simulink model "revLimModel"  (R2017a)
settings: Solver=FixedStepDiscrete  StartTime=0.0  StopTime=3  FixedStep=0.001  RelTol=1e-3
undefined symbols (not defined in the file): GearRatios
libraries: simulink x8
settings Model: Creator=Johnny ZWall  LastModifiedBy=Johnny ZWall
settings DataIOCC: LimitDataPoints=on
settings OptimizationCC: DefaultParameterBehavior=Inlined  UseDivisionForNetSlopeComputation=on  UseFloatMulNetSlope=on  DefaultUnderspecifiedDataType=single  UseSpecifiedMinMax=on  InlineInvariantSignals=on  EnhancedBackFolding=on  CachingGlobalReferences=on  ZeroExternalMemoryAtStartup=off  ZeroInternalMemoryAtStartup=off  NoFixptDivByZeroProtection=on  EfficientFloat2IntCast=on  LifeSpan=inf  OptimizeBlockOrder=speed
settings DebuggingCC: ReadBeforeWriteMsg=EnableAllAsWarning  WriteAfterWriteMsg=EnableAllAsWarning  WriteAfterReadMsg=EnableAllAsWarning  IntegerOverflowMsg=error  UniqueDataStoreMsg=error  AllowSymbolicDim=off  NonBusSignalsTreatedAsBus=error  SFInvalidInputDataAccessInChartInitDiag=error  SFTransitionOutsideNaturalParentDiag=error  SFUnreachableExecutionPathDiag=error  SFUndirectedBroadcastEventsDiag=error  SFExecutionAtInitializationDiag=none  IntegerSaturationMsg=error
settings HardwareCC: ProdBitPerPointer=32  ProdBitPerSizeT=32  ProdBitPerPtrDiffT=32  ProdEndianess=BigEndian  ProdWordSize=32  ProdHWDeviceType=Renesas->SH-2/3/4
settings ModelReferenceCC: ModelReferenceNumInstancesAllowed=Single  PropagateSignalLabelsOutOfModel=off
settings SFSimCC: MATLABDynamicMemAlloc=off
settings RTWCC: SystemTargetFile=ert.tlc  GenCodeOnly=on  TemplateMakefile=ert_default_tmf  Description=Embedded Coder  BuildConfiguration=Faster Runs
settings RTWCC: CustomSourceCode=|
  | #include "EcuHacks.h"
  | 
  | D_Work rtDWork  __attribute__ ((section ("RamHole")));
settings CodeAppCC: GenerateComments=off  IgnoreCustomStorageClasses=off  CustomSymbolStrGlobalVar=rt$N$M  CustomSymbolStrType=$N$M  CustomSymbolStrFcn=$N$M$F  CustomSymbolStrMacro=$N$M  DefineNamingRule=LowerCase  ParamNamingRule=LowerCase  SignalNamingRule=LowerCase  SimulinkBlockComments=off  InternalIdentifier=Classic
settings ERTTargetCC: MultiwordLength=2048  IncludeMdlTerminateFcn=off  CombineSignalStateStructs=on  SuppressErrorStatus=on  SupportAbsoluteTime=off  SupportNonFinite=off  SupportComplex=off  CastingMode=Explicit  ExtModeTransport=2  ExtModeMexFile=sendToCommService  InlinedParameterPlacement=NonHierarchical  MultiInstanceErrorCode=None  RootIOFormat=Structure reference  ERTCustomFileTemplate=example_file_process.tlc  GlobalDataDefinition=InSourceFile  GlobalDataReference=InSourceFile  ERTFilePackagingFormat=Compact  PreserveExpressionOrder=on  PreserveIfCondition=on  IndentStyle=Allman
settings ConfigComp: CovMetricSettings=dw  CovHtmlReporting=on  CovSaveCumulativeToWorkspaceVar=on  CovSaveSingleToWorkspaceVar=on  CovExternalEMLEnable=off

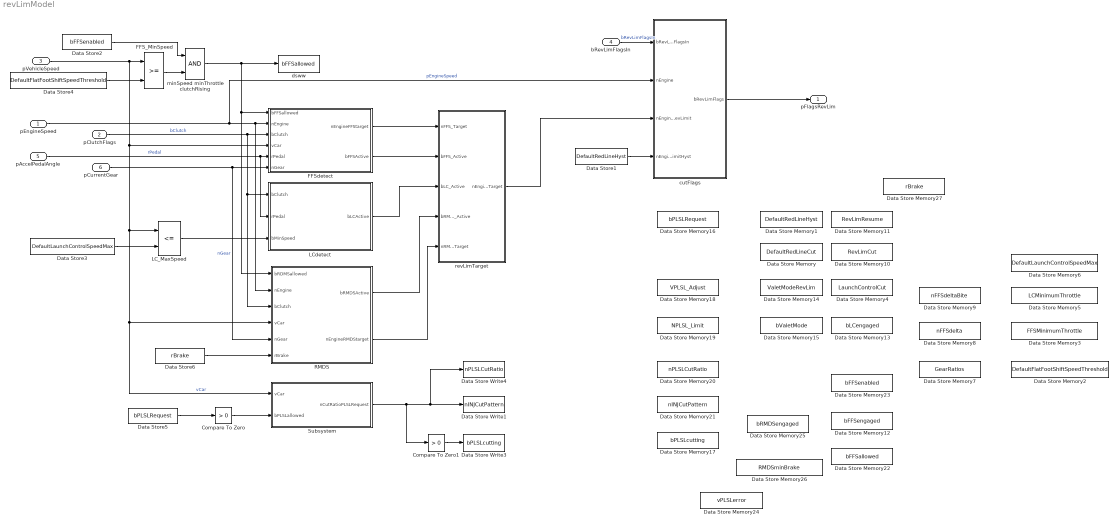
== system revLimModel ==
  pEngineSpeed : Inport  OutDataTypeStr=single  Interpolate=off
  pClutchFlags : Inport  Port=2  OutDataTypeStr=uint8
  pVehicleSpeed : Inport  Port=3  OutDataTypeStr=single
  bRevLimFlagsIn : Inport  Port=4  OutDataTypeStr=uint8
  pAccelPedalAngle : Inport  Port=5  OutDataTypeStr=single
  pCurrentGear : Inport  Port=6  OutDataTypeStr=uint8
  Compare To Zero : simulink/Logic and Bit Operations/Compare To Zero  relop=>  OutDataTypeStr=boolean
  Compare To Zero1 : simulink/Logic and Bit Operations/Compare To Zero  relop=>  OutDataTypeStr=boolean
  Data Store Memory : DataStoreMemory  DataStoreName=DefaultRedLineCut  InitialValue=6700  ShowAdditionalParam=off  OutDataTypeStr=single
  Data Store Memory1 : DataStoreMemory  DataStoreName=DefaultRedLineHyst  ReadBeforeWriteMsg=warning  WriteAfterWriteMsg=error  WriteAfterReadMsg=error  InitialValue=100  ShowAdditionalParam=off  OutDataTypeStr=single
  Data Store Memory10 : DataStoreMemory  DataStoreName=RevLimCut  ReadBeforeWriteMsg=warning  WriteAfterWriteMsg=warning  WriteAfterReadMsg=warning  InitialValue=2500  ShowAdditionalParam=off  OutDataTypeStr=single
  Data Store Memory11 : DataStoreMemory  DataStoreName=RevLimResume  ReadBeforeWriteMsg=warning  WriteAfterWriteMsg=warning  WriteAfterReadMsg=warning  InitialValue=2500  ShowAdditionalParam=off  OutDataTypeStr=single
  Data Store Memory12 : DataStoreMemory  DataStoreName=bFFSengaged  ReadBeforeWriteMsg=warning  WriteAfterWriteMsg=warning  WriteAfterReadMsg=warning  ShowAdditionalParam=off  OutDataTypeStr=boolean
  Data Store Memory13 : DataStoreMemory  DataStoreName=bLCengaged  ReadBeforeWriteMsg=warning  WriteAfterWriteMsg=warning  WriteAfterReadMsg=warning  ShowAdditionalParam=off  OutDataTypeStr=boolean
  Data Store Memory14 : DataStoreMemory  DataStoreName=ValetModeRevLim  InitialValue=4000  ShowAdditionalParam=off  OutDataTypeStr=single
  Data Store Memory15 : DataStoreMemory  DataStoreName=bValetMode  ReadBeforeWriteMsg=warning  WriteAfterWriteMsg=warning  WriteAfterReadMsg=warning  ShowAdditionalParam=off  OutDataTypeStr=uint8
  Data Store Memory16 : DataStoreMemory  DataStoreName=bPLSLRequest  ReadBeforeWriteMsg=warning  WriteAfterWriteMsg=warning  WriteAfterReadMsg=warning  ShowAdditionalParam=off  OutDataTypeStr=boolean
  Data Store Memory17 : DataStoreMemory  DataStoreName=bPLSLcutting  ReadBeforeWriteMsg=warning  WriteAfterWriteMsg=warning  WriteAfterReadMsg=warning  ShowAdditionalParam=off  OutDataTypeStr=boolean
  Data Store Memory18 : DataStoreMemory  DataStoreName=VPLSL_Adjust  ReadBeforeWriteMsg=warning  WriteAfterWriteMsg=warning  WriteAfterReadMsg=warning  ShowAdditionalParam=off  OutDataTypeStr=single
  Data Store Memory19 : DataStoreMemory  DataStoreName=NPLSL_Limit  ReadBeforeWriteMsg=warning  WriteAfterWriteMsg=warning  WriteAfterReadMsg=warning  InitialValue=25  ShowAdditionalParam=off  OutDataTypeStr=single
  Data Store Memory2 : DataStoreMemory  DataStoreName=DefaultFlatFootShiftSpeedThreshold  ReadBeforeWriteMsg=warning  WriteAfterWriteMsg=warning  WriteAfterReadMsg=warning  InitialValue=25  ShowAdditionalParam=off  OutDataTypeStr=single
  Data Store Memory20 : DataStoreMemory  DataStoreName=nPLSLCutRatio  ReadBeforeWriteMsg=warning  WriteAfterWriteMsg=warning  WriteAfterReadMsg=warning  ShowAdditionalParam=off  OutDataTypeStr=uint16
  Data Store Memory21 : DataStoreMemory  DataStoreName=nINJCutPattern  ReadBeforeWriteMsg=warning  WriteAfterWriteMsg=warning  WriteAfterReadMsg=warning  ShowAdditionalParam=off  OutDataTypeStr=uint16
  Data Store Memory22 : DataStoreMemory  DataStoreName=bFFSallowed  ReadBeforeWriteMsg=warning  WriteAfterWriteMsg=warning  WriteAfterReadMsg=warning  ShowAdditionalParam=off  OutDataTypeStr=boolean
  Data Store Memory23 : DataStoreMemory  DataStoreName=bFFSenabled  ReadBeforeWriteMsg=warning  WriteAfterWriteMsg=warning  WriteAfterReadMsg=warning  ShowAdditionalParam=off  OutDataTypeStr=boolean
  Data Store Memory24 : DataStoreMemory  DataStoreName=vPLSLerror  ReadBeforeWriteMsg=warning  WriteAfterWriteMsg=warning  WriteAfterReadMsg=warning  ShowAdditionalParam=off  OutDataTypeStr=single
  Data Store Memory25 : DataStoreMemory  DataStoreName=bRMDSengaged  ReadBeforeWriteMsg=warning  WriteAfterWriteMsg=warning  WriteAfterReadMsg=warning  ShowAdditionalParam=off  OutDataTypeStr=boolean
  Data Store Memory26 : DataStoreMemory  DataStoreName=RMDSminBrake  ReadBeforeWriteMsg=warning  WriteAfterWriteMsg=warning  WriteAfterReadMsg=warning  InitialValue=30  ShowAdditionalParam=off  OutDataTypeStr=single
  Data Store Memory27 : DataStoreMemory  DataStoreName=rBrake  ReadBeforeWriteMsg=warning  WriteAfterWriteMsg=warning  WriteAfterReadMsg=warning  InitialValue=23  ShowAdditionalParam=off  OutDataTypeStr=single
  Data Store Memory3 : DataStoreMemory  DataStoreName=FFSMinimumThrottle  ReadBeforeWriteMsg=warning  WriteAfterWriteMsg=warning  WriteAfterReadMsg=warning  InitialValue=85  ShowAdditionalParam=off  OutDataTypeStr=single
  Data Store Memory4 : DataStoreMemory  DataStoreName=LaunchControlCut  ReadBeforeWriteMsg=warning  WriteAfterWriteMsg=warning  WriteAfterReadMsg=warning  InitialValue=2500  ShowAdditionalParam=off  OutDataTypeStr=single
  Data Store Memory5 : DataStoreMemory  DataStoreName=LCMinimumThrottle  ReadBeforeWriteMsg=warning  WriteAfterWriteMsg=warning  WriteAfterReadMsg=warning  InitialValue=40  ShowAdditionalParam=off  OutDataTypeStr=single
  Data Store Memory6 : DataStoreMemory  DataStoreName=DefaultLaunchControlSpeedMax  ReadBeforeWriteMsg=warning  WriteAfterWriteMsg=warning  WriteAfterReadMsg=warning  InitialValue=3  ShowAdditionalParam=off  OutDataTypeStr=single
  Data Store Memory7 : DataStoreMemory  DataStoreName=GearRatios  ReadBeforeWriteMsg=warning  WriteAfterWriteMsg=warning  WriteAfterReadMsg=warning  InitialValue=[3.636,2.235,1.521,1.137,0.971,0.756]  ShowAdditionalParam=off  OutDataTypeStr=single  Dimensions=6
  Data Store Memory8 : DataStoreMemory  DataStoreName=nFFSdelta  ReadBeforeWriteMsg=warning  WriteAfterWriteMsg=warning  WriteAfterReadMsg=warning  InitialValue=300  ShowAdditionalParam=off  OutDataTypeStr=single
  Data Store Memory9 : DataStoreMemory  DataStoreName=nFFSdeltaBite  ReadBeforeWriteMsg=warning  WriteAfterWriteMsg=warning  WriteAfterReadMsg=warning  InitialValue=100  ShowAdditionalParam=off  OutDataTypeStr=single
  Data Store Write1 : DataStoreWrite  DataStoreName=nINJCutPattern
  Data Store Write3 : DataStoreWrite  DataStoreName=bPLSLcutting
  Data Store Write4 : DataStoreWrite  DataStoreName=nPLSLCutRatio
  Data Store1 : DataStoreRead  DataStoreName=DefaultRedLineHyst
  Data Store2 : DataStoreRead  DataStoreName=bFFSenabled  DataStoreElements=bFFSenabled
  Data Store3 : DataStoreRead  DataStoreName=DefaultLaunchControlSpeedMax
  Data Store4 : DataStoreRead  DataStoreName=DefaultFlatFootShiftSpeedThreshold
  Data Store5 : DataStoreRead  DataStoreName=bPLSLRequest  DataStoreElements=bPLSLRequest
  Data Store6 : DataStoreRead  DataStoreName=rBrake  DataStoreElements=rBrake
  FFS_MinSpeed : RelationalOperator  OutDataTypeStr=boolean  RndMeth=Nearest
  FFSdetect : Subsystem
  LC_MaxSpeed : RelationalOperator  Operator=<=  OutDataTypeStr=boolean  RndMeth=Nearest
  LCdetect : Subsystem
  RMDS : Subsystem
  Subsystem : Subsystem
  cutFlags : Subsystem
  dsww : DataStoreWrite  DataStoreName=bFFSallowed
  minSpeed minThrottle clutchRising : Logic  AllPortsSameDT=off  OutDataTypeStr=boolean
  revLimTarget : Subsystem
  pFlagsRevLim : Outport  SignalName=pFlagsRevLim  OutDataTypeStr=uint8
  wires:
  cutFlags/1(bRevLimFlags) -> pFlagsRevLim/1
  revLimTarget/1(nEngineTarget) -> cutFlags/3(nEngineRevLimit)
  pVehicleSpeed/1 -> FFSdetect/4(vCar), LC_MaxSpeed/1, RMDS/4(vCar), Subsystem/1(vCar), FFS_MinSpeed/1  "vCar"
  LC_MaxSpeed/1 -> LCdetect/3(bMinSpeed)
  minSpeed minThrottle clutchRising/1 -> dsww/1, FFSdetect/1(bFFSallowed), RMDS/1(bRDMSallowed)
  Data Store3/1 -> LC_MaxSpeed/2
  pCurrentGear/1 -> RMDS/5(nGear), FFSdetect/6(nGear)  "nGear"
  pAccelPedalAngle/1 -> LCdetect/2(rPedal), FFSdetect/5(rPedal)  "rPedal"
  Data Store4/1 -> FFS_MinSpeed/2
  Data Store1/1 -> cutFlags/4(nEngineCutLimitHyst)
  pClutchFlags/1 -> RMDS/3(bClutch), LCdetect/1(bClutch), FFSdetect/3(bClutch)  "bClutch"
  bRevLimFlagsIn/1 -> cutFlags/1(bRevLimFlagsIn)  "bRevLimFlagsIn"
  pEngineSpeed/1 -> cutFlags/2(nEngine), RMDS/2(nEngine), FFSdetect/2(nEngine)  "pEngineSpeed"
  FFSdetect/1(nEngineFFStarget) -> revLimTarget/1(nFFS_Target)
  FFSdetect/2(bFFSActive) -> revLimTarget/2(bFFS_Active)
  LCdetect/1(bLCActive) -> revLimTarget/3(bLC_Active)
  Data Store5/1 -> Compare To Zero/1
  Compare To Zero/1 -> Subsystem/2(bPLSLallowed)
  FFS_MinSpeed/1 -> minSpeed minThrottle clutchRising/2
  Data Store2/1 -> minSpeed minThrottle clutchRising/1
  Compare To Zero1/1 -> Data Store Write3/1
  Subsystem/1(nCutRatioPLSLRequest) -> Data Store Write4/1, Data Store Write1/1, Compare To Zero1/1
  Data Store6/1 -> RMDS/6(rBrake)
  RMDS/1(bRMDSActive) -> revLimTarget/4(bRMDS_Active)
  RMDS/2(nEngineRMDStarget) -> revLimTarget/5(nRMDS_Target)

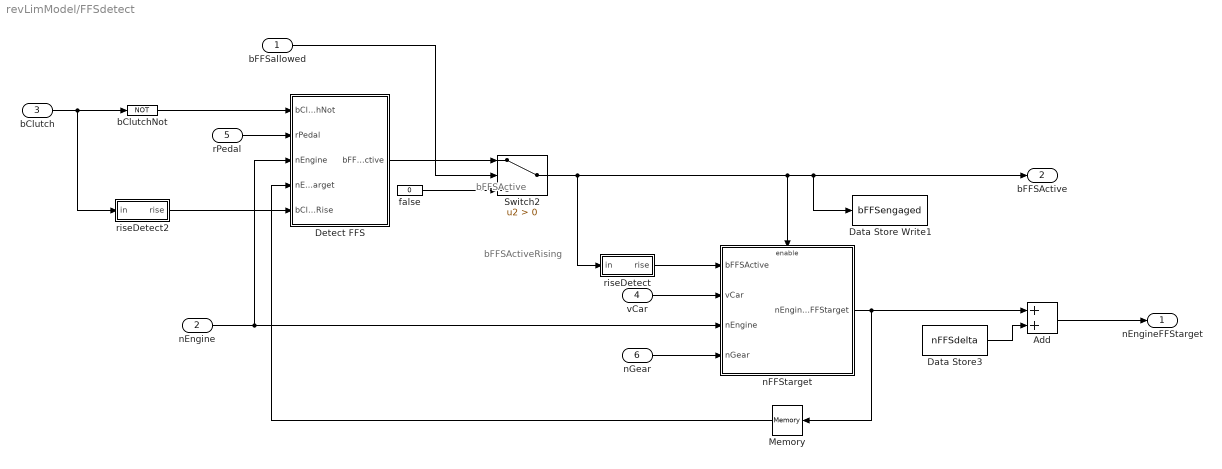
== system revLimModel/FFSdetect ==
  note: bFFSActiveRising
  note: bFFSActive
  bFFSallowed : Inport
  nEngine : Inport  Port=2
  bClutch : Inport  Port=3
  vCar : Inport  Port=4
  rPedal : Inport  Port=5
  nGear : Inport  Port=6
  Add : Sum
  Data Store Write1 : DataStoreWrite  DataStoreName=bFFSengaged
  Data Store3 : DataStoreRead  DataStoreName=nFFSdelta
  Detect FFS : Subsystem
  Memory : Memory
  Switch2 : Switch  Criteria=u2 > Threshold
  bClutchNot : Logic  Operator=NOT  AllPortsSameDT=off  OutDataTypeStr=boolean
  false : Constant  Value=0  OutDataTypeStr=boolean
  nFFStarget : Subsystem
      settings: RTWSystemCode=Inline
  riseDetect : Subsystem
  riseDetect2 : Subsystem
  nEngineFFStarget : Outport  InitialOutput=[0]
  bFFSActive : Outport  Port=2  OutputWhenDisabled=reset  InitialOutput=[0]
  wires:
  vCar/1 -> nFFStarget/2(vCar)
  nEngine/1 -> Detect FFS/3(nEngine), nFFStarget/3(nEngine)
  nGear/1 -> nFFStarget/4(nGear)
  nFFStarget/1(nEngineFFStarget) -> Memory/1, Add/1
  bClutch/1 -> bClutchNot/1, riseDetect2/1(in)
  rPedal/1 -> Detect FFS/2(rPedal)
  Switch2/1 -> riseDetect/1(in), Data Store Write1/1, bFFSActive/1, nFFStarget/Enable
  riseDetect/1(rise) -> nFFStarget/1(bFFSActive)
  Add/1 -> nEngineFFStarget/1
  Data Store3/1 -> Add/2
  Memory/1 -> Detect FFS/4(nEngineFFStarget)
  riseDetect2/1(rise) -> Detect FFS/5(bClutchRise)
  bClutchNot/1 -> Detect FFS/1(bClutchNot)
  Detect FFS/1(bFFSActive) -> Switch2/1
  bFFSallowed/1 -> Switch2/2
  false/1 -> Switch2/3

== system revLimModel/LCdetect ==
  bClutch : Inport
  rPedal : Inport  Port=2
  bMinSpeed : Inport  Port=3
  Data Store3 : DataStoreRead  DataStoreName=LCMinimumThrottle
  LC_MinPedal : RelationalOperator  OutDataTypeStr=boolean  RndMeth=Nearest
  maxSpeed minThrottle clutchRising : Logic  Inputs=3  AllPortsSameDT=off  OutDataTypeStr=boolean
  bLCActive : Outport  OutputWhenDisabled=reset  InitialOutput=[0]
  wires:
  Data Store3/1 -> LC_MinPedal/2
  rPedal/1 -> LC_MinPedal/1
  maxSpeed minThrottle clutchRising/1 -> bLCActive/1  "bLCstateSet"
  LC_MinPedal/1 -> maxSpeed minThrottle clutchRising/3  "bLCrPedakOK"
  bClutch/1 -> maxSpeed minThrottle clutchRising/2  "bClutchFalling"
  bMinSpeed/1 -> maxSpeed minThrottle clutchRising/1

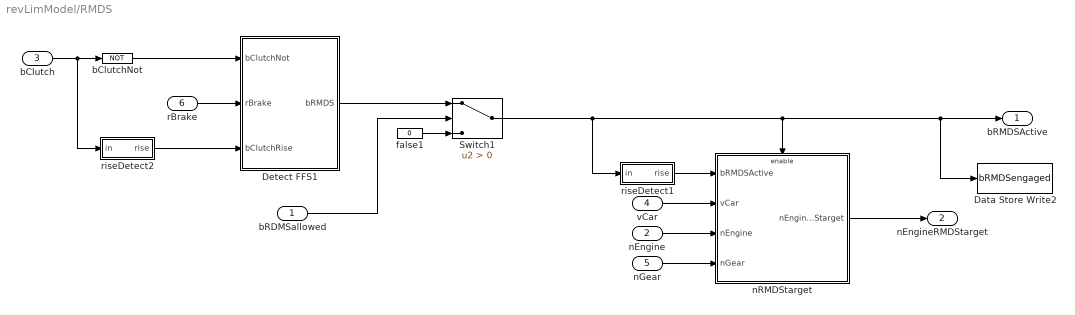
== system revLimModel/RMDS ==
  bRDMSallowed : Inport
  nEngine : Inport  Port=2
  bClutch : Inport  Port=3
  vCar : Inport  Port=4
  nGear : Inport  Port=5
  rBrake : Inport  Port=6
  Data Store Write2 : DataStoreWrite  DataStoreName=bRMDSengaged
  Detect FFS1 : Subsystem
  Switch1 : Switch  Criteria=u2 > Threshold
  bClutchNot : Logic  Operator=NOT  AllPortsSameDT=off  OutDataTypeStr=boolean
  false1 : Constant  Value=0  OutDataTypeStr=boolean
  nRMDStarget : Subsystem
      settings: RTWSystemCode=Inline
  riseDetect1 : Subsystem
  riseDetect2 : Subsystem
  bRMDSActive : Outport  OutputWhenDisabled=reset  InitialOutput=[0]
  nEngineRMDStarget : Outport  Port=2  InitialOutput=[0]
  wires:
  vCar/1 -> nRMDStarget/2(vCar)
  nEngine/1 -> nRMDStarget/3(nEngine)
  nGear/1 -> nRMDStarget/4(nGear)
  bClutch/1 -> bClutchNot/1, riseDetect2/1(in)
  rBrake/1 -> Detect FFS1/2(rBrake)
  Switch1/1 -> Data Store Write2/1, bRMDSActive/1, nRMDStarget/Enable, riseDetect1/1(in)
  nRMDStarget/1(nEngineRMDStarget) -> nEngineRMDStarget/1
  riseDetect1/1(rise) -> nRMDStarget/1(bRMDSActive)
  riseDetect2/1(rise) -> Detect FFS1/3(bClutchRise)
  bClutchNot/1 -> Detect FFS1/1(bClutchNot)
  Detect FFS1/1(bRMDS) -> Switch1/1
  bRDMSallowed/1 -> Switch1/2
  false1/1 -> Switch1/3

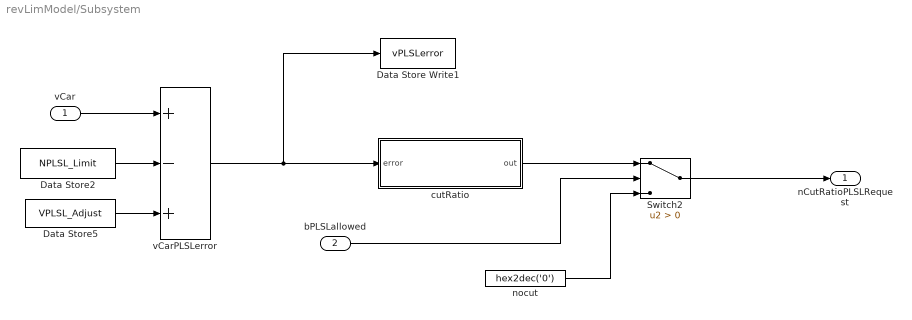
== system revLimModel/Subsystem ==
  vCar : Inport
  bPLSLallowed : Inport  Port=2
  Data Store Write1 : DataStoreWrite  DataStoreName=vPLSLerror  DataStoreElements=vPLSLerror
  Data Store2 : DataStoreRead  DataStoreName=NPLSL_Limit
  Data Store5 : DataStoreRead  DataStoreName=VPLSL_Adjust  DataStoreElements=VPLSL_Adjust
  Switch2 : Switch  Criteria=u2 > Threshold
  cutRatio : Subsystem
  nocut : Constant  Value=hex2dec('0')  OutDataTypeStr=uint16
  vCarPLSLerror : Sum  Inputs=+-+
  nCutRatioPLSLRequest : Outport  OutDataTypeStr=uint16  OutputWhenDisabled=reset  InitialOutput=[0]
  wires:
  Data Store2/1 -> vCarPLSLerror/2
  vCar/1 -> vCarPLSLerror/1
  Data Store5/1 -> vCarPLSLerror/3
  vCarPLSLerror/1 -> Data Store Write1/1, cutRatio/1(error)
  cutRatio/1(out) -> Switch2/1
  Switch2/1 -> nCutRatioPLSLRequest/1
  bPLSLallowed/1 -> Switch2/2
  nocut/1 -> Switch2/3

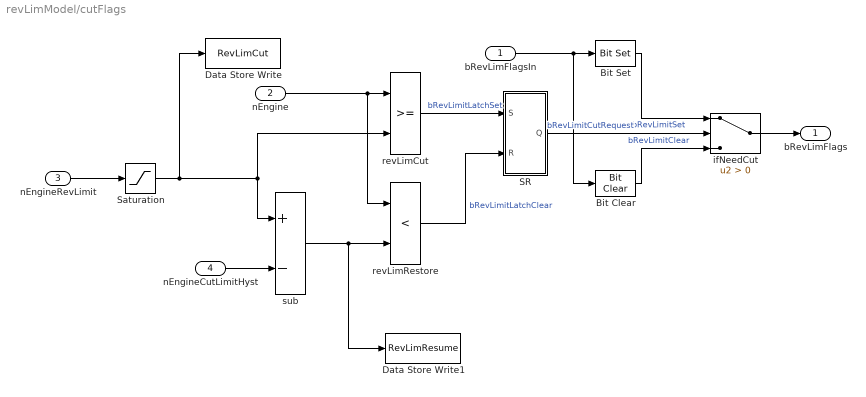
== system revLimModel/cutFlags ==
  bRevLimFlagsIn : Inport  OutDataTypeStr=uint8
  nEngine : Inport  Port=2
  nEngineRevLimit : Inport  Port=3
  nEngineCutLimitHyst : Inport  Port=4
  Bit Clear : simulink/Logic and Bit Operations/Bit Clear  iBit=0
      settings: SourceProductName=Simulink  SourceProductBaseCode=SL
  Bit Set : simulink/Logic and Bit Operations/Bit Set  iBit=0
      settings: SourceProductName=Simulink  SourceProductBaseCode=SL
  Data Store Write : DataStoreWrite  DataStoreName=RevLimCut
  Data Store Write1 : DataStoreWrite  DataStoreName=RevLimResume
  SR : Subsystem
  Saturation : Saturate  UpperLimit=6800  LowerLimit=2100
  ifNeedCut : Switch  Criteria=u2 > Threshold
  revLimCut : RelationalOperator  OutDataTypeStr=boolean  RndMeth=Nearest
  revLimRestore : RelationalOperator  Operator=<  OutDataTypeStr=boolean  RndMeth=Nearest
  sub : Sum  Inputs=+-
  bRevLimFlags : Outport
  wires:
  Bit Clear/1 -> ifNeedCut/3  "bRevLimitClear"
  nEngineCutLimitHyst/1 -> sub/2
  nEngine/1 -> revLimRestore/1, revLimCut/1
  sub/1 -> Data Store Write1/1, revLimRestore/2
  ifNeedCut/1 -> bRevLimFlags/1
  revLimCut/1 -> SR/1(S)  "bRevLimitLatchSet"
  bRevLimFlagsIn/1 -> Bit Clear/1, Bit Set/1
  revLimRestore/1 -> SR/2(R)  "bRevLimitLatchClear"
  Bit Set/1 -> ifNeedCut/1  "bRevLimitSet"
  SR/1(Q) -> ifNeedCut/2  "bRevLimitCutRequest"
  Saturation/1 -> Data Store Write/1, sub/1, revLimCut/2
  nEngineRevLimit/1 -> Saturation/1

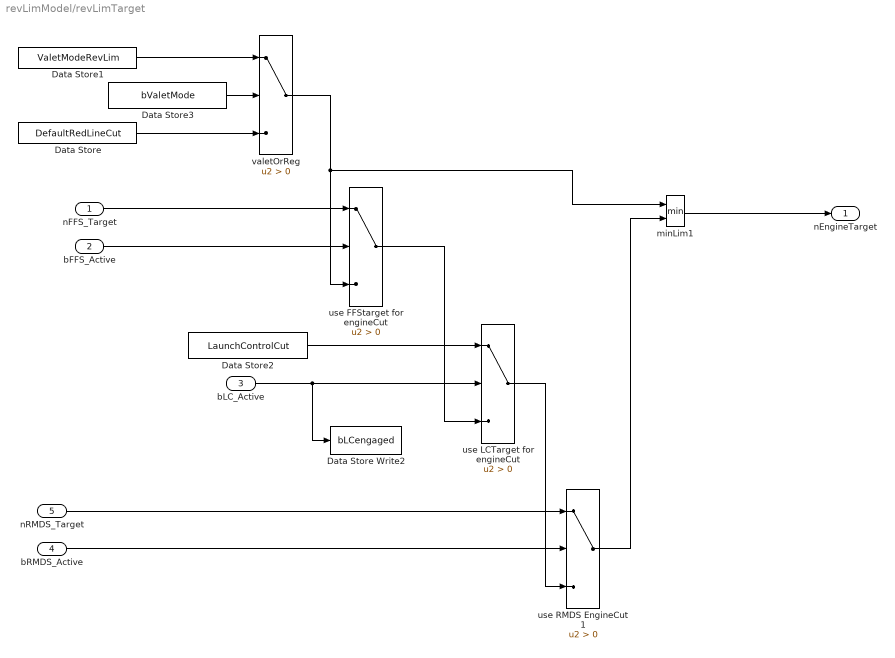
== system revLimModel/revLimTarget ==
  nFFS_Target : Inport
  bFFS_Active : Inport  Port=2
  bLC_Active : Inport  Port=3
  bRMDS_Active : Inport  Port=4
  nRMDS_Target : Inport  Port=5
  Data Store : DataStoreRead  DataStoreName=DefaultRedLineCut
  Data Store Write2 : DataStoreWrite  DataStoreName=bLCengaged
  Data Store1 : DataStoreRead  DataStoreName=ValetModeRevLim
  Data Store2 : DataStoreRead  DataStoreName=LaunchControlCut  DataStoreElements=LaunchControlCut
  Data Store3 : DataStoreRead  DataStoreName=bValetMode  DataStoreElements=bValetMode
  minLim1 : MinMax  Inputs=2  OutDataTypeStr=single
  use FFStarget for engineCut : Switch  Criteria=u2 > Threshold  OutDataTypeStr=single
  use LCTarget for engineCut : Switch  Criteria=u2 > Threshold  OutDataTypeStr=single
  use RMDS EngineCut1 : Switch  Criteria=u2 > Threshold  OutDataTypeStr=single
  valetOrReg : Switch  Criteria=u2 > Threshold  OutDataTypeStr=single
  nEngineTarget : Outport
  wires:
  bLC_Active/1 -> Data Store Write2/1, use LCTarget for engineCut/2
  use RMDS EngineCut1/1 -> minLim1/2
  bFFS_Active/1 -> use FFStarget for engineCut/2
  valetOrReg/1 -> minLim1/1, use FFStarget for engineCut/3
  use FFStarget for engineCut/1 -> use LCTarget for engineCut/3
  Data Store2/1 -> use LCTarget for engineCut/1
  nFFS_Target/1 -> use FFStarget for engineCut/1
  minLim1/1 -> nEngineTarget/1
  Data Store/1 -> valetOrReg/3
  Data Store1/1 -> valetOrReg/1
  Data Store3/1 -> valetOrReg/2
  nRMDS_Target/1 -> use RMDS EngineCut1/1
  bRMDS_Active/1 -> use RMDS EngineCut1/2
  use LCTarget for engineCut/1 -> use RMDS EngineCut1/3

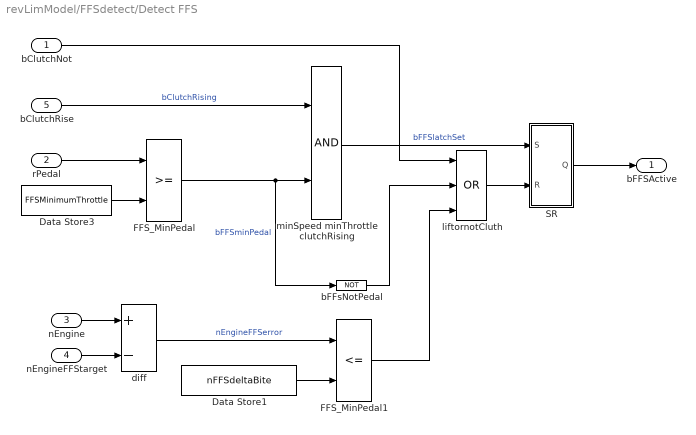
== system revLimModel/FFSdetect/Detect FFS ==
  bClutchNot : Inport
  rPedal : Inport  Port=2
  nEngine : Inport  Port=3
  nEngineFFStarget : Inport  Port=4
  bClutchRise : Inport  Port=5
  Data Store1 : DataStoreRead  DataStoreName=nFFSdeltaBite
  Data Store3 : DataStoreRead  DataStoreName=FFSMinimumThrottle
  FFS_MinPedal : RelationalOperator  OutDataTypeStr=boolean  RndMeth=Nearest
  FFS_MinPedal1 : RelationalOperator  Operator=<=  OutDataTypeStr=boolean  RndMeth=Nearest
  SR : Subsystem
  bFFsNotPedal : Logic  Operator=NOT  AllPortsSameDT=off  OutDataTypeStr=boolean
  diff : Sum  Inputs=+-
  "liftornotCluth " : Logic  Operator=OR  Inputs=3  AllPortsSameDT=off  OutDataTypeStr=boolean
  minSpeed minThrottle clutchRising : Logic  AllPortsSameDT=off  OutDataTypeStr=boolean
  bFFSActive : Outport
  wires:
  Data Store3/1 -> FFS_MinPedal/2
  rPedal/1 -> FFS_MinPedal/1
  bClutchRise/1 -> minSpeed minThrottle clutchRising/1  "bClutchRising"
  SR/1(Q) -> bFFSActive/1
  minSpeed minThrottle clutchRising/1 -> SR/1(S)  "bFFSlatchSet"
  FFS_MinPedal/1 -> bFFsNotPedal/1, minSpeed minThrottle clutchRising/2  "bFFSminPedal"
  bClutchNot/1 -> "liftornotCluth "/1
  "liftornotCluth "/1 -> SR/2(R)
  bFFsNotPedal/1 -> "liftornotCluth "/2
  nEngine/1 -> diff/1
  nEngineFFStarget/1 -> diff/2
  diff/1 -> FFS_MinPedal1/1  "nEngineFFSerror"
  Data Store1/1 -> FFS_MinPedal1/2
  FFS_MinPedal1/1 -> "liftornotCluth "/3

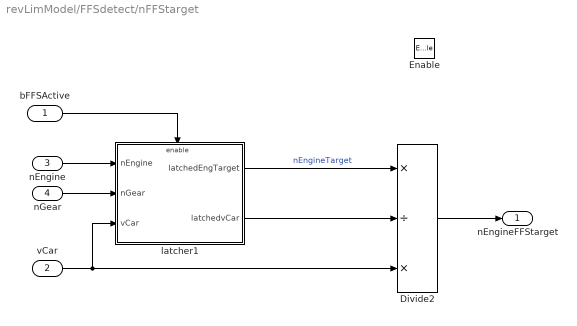
== system revLimModel/FFSdetect/nFFStarget ==
  bFFSActive : Inport
  vCar : Inport  Port=2
  nEngine : Inport  Port=3
  nGear : Inport  Port=4
  Enable : EnablePort
  Divide2 : Product  Inputs=*/*
  latcher1 : Subsystem
  nEngineFFStarget : Outport
  wires:
  Divide2/1 -> nEngineFFStarget/1
  vCar/1 -> Divide2/3, latcher1/3(vCar)
  latcher1/1(latchedEngTarget) -> Divide2/1  "nEngineTarget"
  bFFSActive/1 -> latcher1/Enable
  nGear/1 -> latcher1/2(nGear)
  latcher1/2(latchedvCar) -> Divide2/2
  nEngine/1 -> latcher1/1(nEngine)

== system revLimModel/FFSdetect/riseDetect ==
  in : Inport
  Memory : Memory
  rising : RelationalOperator  Operator=>  OutDataTypeStr=boolean  RndMeth=Simplest
  rise : Outport
  wires:
  Memory/1 -> rising/2
  in/1 -> rising/1, Memory/1
  rising/1 -> rise/1

== system revLimModel/FFSdetect/riseDetect2 ==
  in : Inport
  Memory : Memory
  rising : RelationalOperator  Operator=>  OutDataTypeStr=boolean  RndMeth=Simplest
  rise : Outport
  wires:
  Memory/1 -> rising/2
  in/1 -> rising/1, Memory/1
  rising/1 -> rise/1

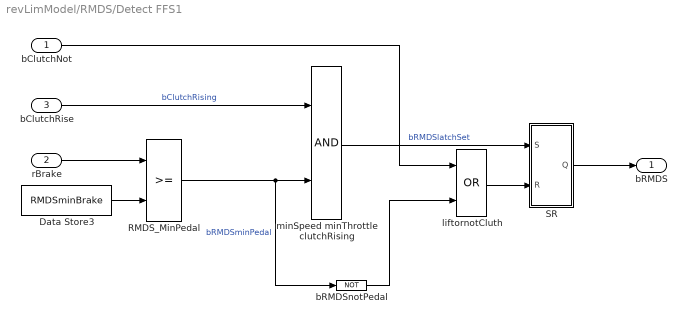
== system revLimModel/RMDS/Detect FFS1 ==
  bClutchNot : Inport
  rBrake : Inport  Port=2
  bClutchRise : Inport  Port=3
  Data Store3 : DataStoreRead  DataStoreName=RMDSminBrake
  RMDS_MinPedal : RelationalOperator  OutDataTypeStr=boolean  RndMeth=Nearest
  SR : Subsystem
  bRMDSnotPedal : Logic  Operator=NOT  AllPortsSameDT=off  OutDataTypeStr=boolean
  "liftornotCluth " : Logic  Operator=OR  AllPortsSameDT=off  OutDataTypeStr=boolean
  minSpeed minThrottle clutchRising : Logic  AllPortsSameDT=off  OutDataTypeStr=boolean
  bRMDS : Outport
  wires:
  Data Store3/1 -> RMDS_MinPedal/2
  rBrake/1 -> RMDS_MinPedal/1
  bClutchRise/1 -> minSpeed minThrottle clutchRising/1  "bClutchRising"
  SR/1(Q) -> bRMDS/1
  minSpeed minThrottle clutchRising/1 -> SR/1(S)  "bRMDSlatchSet"
  RMDS_MinPedal/1 -> bRMDSnotPedal/1, minSpeed minThrottle clutchRising/2  "bRMDSminPedal"
  bClutchNot/1 -> "liftornotCluth "/1
  "liftornotCluth "/1 -> SR/2(R)
  bRMDSnotPedal/1 -> "liftornotCluth "/2

== system revLimModel/RMDS/nRMDStarget ==
  bRMDSActive : Inport
  vCar : Inport  Port=2
  nEngine : Inport  Port=3
  nGear : Inport  Port=4
  Enable : EnablePort
  Divide2 : Product  Inputs=*/*
  latcher1 : Subsystem
  nEngineRMDStarget : Outport
  wires:
  Divide2/1 -> nEngineRMDStarget/1
  vCar/1 -> Divide2/3, latcher1/3(vCar)
  latcher1/1(latchedEngTarget) -> Divide2/1  "nEngineTarget"
  bRMDSActive/1 -> latcher1/Enable
  nGear/1 -> latcher1/2(nGear)
  latcher1/2(latchedvCar) -> Divide2/2
  nEngine/1 -> latcher1/1(nEngine)

== system revLimModel/RMDS/riseDetect1 ==
  in : Inport
  Memory : Memory
  rising : RelationalOperator  Operator=>  OutDataTypeStr=boolean  RndMeth=Simplest
  rise : Outport
  wires:
  Memory/1 -> rising/2
  in/1 -> rising/1, Memory/1
  rising/1 -> rise/1

== system revLimModel/RMDS/riseDetect2 ==
  in : Inport
  Memory : Memory
  rising : RelationalOperator  Operator=>  OutDataTypeStr=boolean  RndMeth=Simplest
  rise : Outport
  wires:
  Memory/1 -> rising/2
  in/1 -> rising/1, Memory/1
  rising/1 -> rise/1

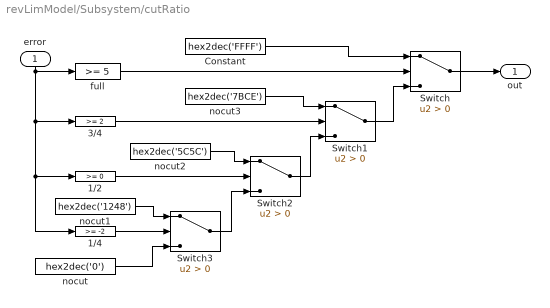
== system revLimModel/Subsystem/cutRatio ==
  error : Inport
  1/2 : simulink/Logic and Bit Operations/Compare To Constant  relop=>=  const=0  OutDataTypeStr=boolean
  1/4 : simulink/Logic and Bit Operations/Compare To Constant  relop=>=  const=-2  OutDataTypeStr=boolean
  3/4 : simulink/Logic and Bit Operations/Compare To Constant  relop=>=  const=2  OutDataTypeStr=boolean
  Constant : Constant  Value=hex2dec('FFFF')  OutDataTypeStr=uint16
  Switch{,1..3} (4 alike) : Switch  Criteria=u2 > Threshold
  full : simulink/Logic and Bit Operations/Compare To Constant  relop=>=  const=5  OutDataTypeStr=boolean
  nocut : Constant  Value=hex2dec('0')  OutDataTypeStr=uint16
  nocut1 : Constant  Value=hex2dec('1248')  OutDataTypeStr=uint16
  nocut2 : Constant  Value=hex2dec('5C5C')  OutDataTypeStr=uint16
  nocut3 : Constant  Value=hex2dec('7BCE')  OutDataTypeStr=uint16
  out : Outport
  wires:
  nocut1/1 -> Switch3/1
  1/2/1 -> Switch2/2
  Switch2/1 -> Switch1/3
  1/4/1 -> Switch3/2
  3/4/1 -> Switch1/2
  Switch/1 -> out/1
  full/1 -> Switch/2
  Switch3/1 -> Switch2/3
  error/1 -> full/1, 3/4/1, 1/2/1, 1/4/1
  nocut/1 -> Switch3/3
  nocut3/1 -> Switch1/1
  Switch1/1 -> Switch/3
  Constant/1 -> Switch/1
  nocut2/1 -> Switch2/1

== system revLimModel/cutFlags/SR ==
  S : Inport
  R : Inport  Port=2
  mem : Memory
  notMem : Logic  Operator=NOT  AllPortsSameDT=off  OutDataTypeStr=boolean
  reset : Logic  Operator=NOR  AllPortsSameDT=off  OutDataTypeStr=boolean
  set : Logic  Operator=OR  AllPortsSameDT=off  OutDataTypeStr=boolean
  Q : Outport
  wires:
  S/1 -> set/1
  set/1 -> mem/1, Q/1
  reset/1 -> set/2
  mem/1 -> notMem/1
  notMem/1 -> reset/1
  R/1 -> reset/2

== system revLimModel/FFSdetect/Detect FFS/SR ==
  S : Inport
  R : Inport  Port=2
  mem : Memory
  notMem : Logic  Operator=NOT  AllPortsSameDT=off  OutDataTypeStr=boolean
  reset : Logic  Operator=NOR  AllPortsSameDT=off  OutDataTypeStr=boolean
  set : Logic  Operator=OR  AllPortsSameDT=off  OutDataTypeStr=boolean
  Q : Outport
  wires:
  S/1 -> set/1
  set/1 -> mem/1, Q/1
  reset/1 -> set/2
  mem/1 -> notMem/1
  notMem/1 -> reset/1
  R/1 -> reset/2

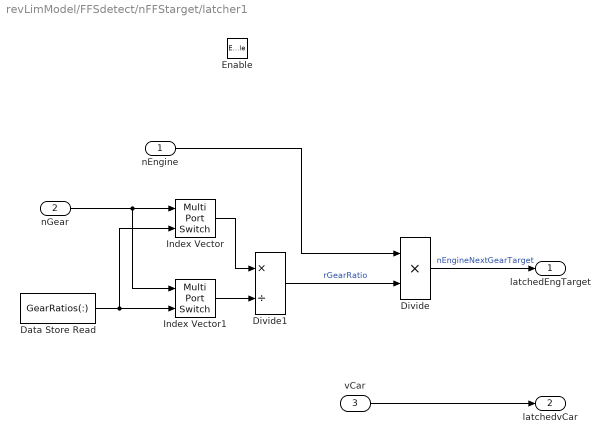
== system revLimModel/FFSdetect/nFFStarget/latcher1 ==
  nEngine : Inport
  nGear : Inport  Port=2
  vCar : Inport  Port=3
  Enable : EnablePort
  Data Store Read : DataStoreRead  DataStoreName=GearRatios  DataStoreElements=GearRatios(:)
  Divide : Product  Inputs=**
  Divide1 : Product  Inputs=*/
  Index Vector : MultiPortSwitch  DataPortOrder=Zero-based contiguous  Inputs=1  zeroidx=on
  Index Vector1 : MultiPortSwitch  Inputs=1
  latchedEngTarget : Outport
  latchedvCar : Outport  Port=2
  wires:
  Divide/1 -> latchedEngTarget/1  "nEngineNextGearTarget"
  nEngine/1 -> Divide/1
  Divide1/1 -> Divide/2  "rGearRatio"
  nGear/1 -> Index Vector1/1, Index Vector/1
  vCar/1 -> latchedvCar/1
  Data Store Read/1 -> Index Vector/2, Index Vector1/2
  Index Vector/1 -> Divide1/1
  Index Vector1/1 -> Divide1/2

== system revLimModel/RMDS/Detect FFS1/SR ==
  S : Inport
  R : Inport  Port=2
  mem : Memory
  notMem : Logic  Operator=NOT  AllPortsSameDT=off  OutDataTypeStr=boolean
  reset : Logic  Operator=NOR  AllPortsSameDT=off  OutDataTypeStr=boolean
  set : Logic  Operator=OR  AllPortsSameDT=off  OutDataTypeStr=boolean
  Q : Outport
  wires:
  S/1 -> set/1
  set/1 -> mem/1, Q/1
  reset/1 -> set/2
  mem/1 -> notMem/1
  notMem/1 -> reset/1
  R/1 -> reset/2

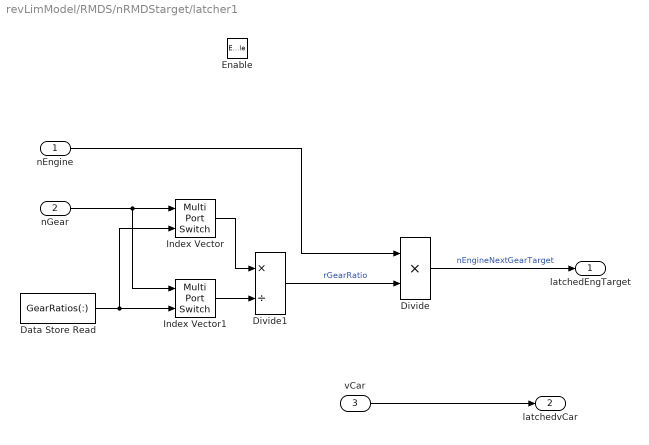
== system revLimModel/RMDS/nRMDStarget/latcher1 ==
  nEngine : Inport
  nGear : Inport  Port=2
  vCar : Inport  Port=3
  Enable : EnablePort
  Data Store Read : DataStoreRead  DataStoreName=GearRatios  DataStoreElements=GearRatios(:)
  Divide : Product  Inputs=**
  Divide1 : Product  Inputs=*/
  Index Vector : MultiPortSwitch  Inputs=1
  Index Vector1 : MultiPortSwitch  DataPortOrder=Zero-based contiguous  Inputs=1
  latchedEngTarget : Outport
  latchedvCar : Outport  Port=2
  wires:
  Divide/1 -> latchedEngTarget/1  "nEngineNextGearTarget"
  nEngine/1 -> Divide/1
  Divide1/1 -> Divide/2  "rGearRatio"
  nGear/1 -> Index Vector1/1, Index Vector/1
  vCar/1 -> latchedvCar/1
  Data Store Read/1 -> Index Vector/2, Index Vector1/2
  Index Vector/1 -> Divide1/1
  Index Vector1/1 -> Divide1/2
